simulink model "compile"  (R2021b)
settings: Solver=VariableStepAuto  StartTime=0.0  StopTime=10.0  RelTol=1e-3
settings Model: Creator=delur  LastModifiedBy=delur

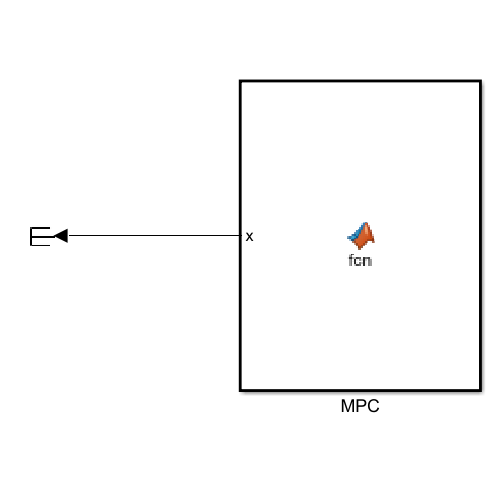
[thumbnail: Simulink's stored preview of the top-level diagram]
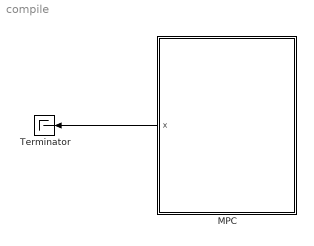
== system compile ==
  MPC : MATLAB Function  TreatAsAtomicUnit=on
  Terminator : Terminator
  wires:
  MPC/1(x) -> Terminator/1

== matlab function compile/MPC ==
  data: x output
function x = fcn()
x = run_cvx;
end
